simulink model "cascadedSubsystem_filter"  (R2020a)
settings: Solver=VariableStepAuto  StartTime=0.0  StopTime=10.0  RelTol=1e-3
settings Model: Creator=DELL  LastModifiedBy=DELL
settings DataIOCC: SaveOutput=off  SaveTime=off

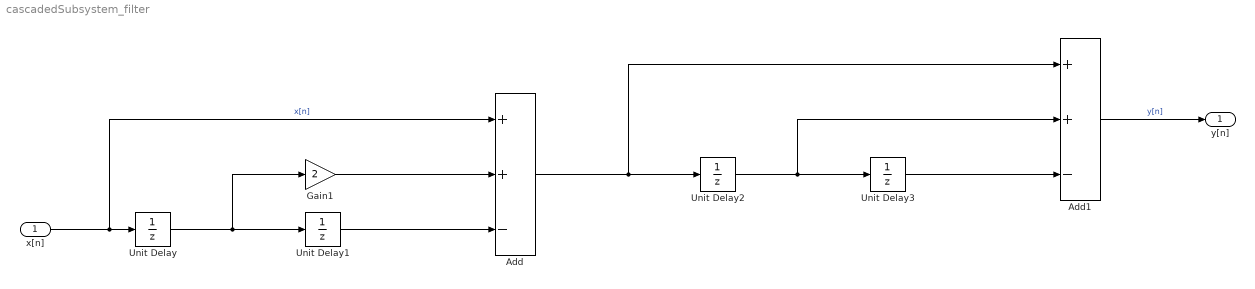
== system cascadedSubsystem_filter ==
  x[n] : Inport  OutDataTypeStr=double  PortDimensions=1  SampleTime=[0,1]
  Add : Sum  Inputs=++-
  Add1 : Sum  Inputs=++-
  Gain1 : Gain  Gain=2
  Unit Delay{,1..3} (4 alike) : UnitDelay  SampleTime=-1  HasFrameUpgradeWarning=on
  y[n] : Outport  OutDataTypeStr=double  PortDimensions=1  SampleTime=[0,1]
  wires:
  Unit Delay2/1 -> Unit Delay3/1, Add1/2
  Unit Delay/1 -> Unit Delay1/1, Gain1/1
  x[n]/1 -> Unit Delay/1, Add/1  "x[n]"
  Gain1/1 -> Add/2
  Add/1 -> Unit Delay2/1, Add1/1
  Unit Delay3/1 -> Add1/3
  Unit Delay1/1 -> Add/3
  Add1/1 -> y[n]/1  "y[n]"
